simulink model "ModelOfTheRocket"  (R2020b)
settings: Solver=ode45  StartTime=0.0  StopTime=10  RelTol=1e-5
PostLoadFcn:
  | flightControlCallback('initializeParameters', bdroot, '3DOF', 0);
InitFcn:
  | flightControlCallback('runSim', bdroot);
libraries: aerolibasang x2, shared3dof x1, aerolibanim x1, simulink_extras x1
settings Model: Creator=yudan  LastModifiedBy=yudan
settings SolverCC: MinimalZcImpactIntegration=on
settings DataIOCC: ExternalInput=getinputstruct(op);  InitialState=getstatestruct(op);  SaveFormat=Array
settings OptimizationCC: EnhancedBackFolding=on  StrengthReduction=on  InitFltsAndDblsToZero=on  DifferentSizesBufferReuse=on
settings DebuggingCC: WriteAfterWriteMsg=DisableAll  AlgebraicLoopMsg=none  FcnCallInpInsideContextMsg=warning  UnconnectedInputMsg=none  UnconnectedOutputMsg=none  UnconnectedLineMsg=none  UniqueDataStoreMsg=error  StateNameClashWarn=warning  StrictBusMsg=ErrorOnBusTreatedAsVector  SFUnexpectedBacktrackingDiag=warning  SFNoUnconditionalDefaultTransitionDiag=warning  SFExecutionAtInitializationDiag=none  ArithmeticOperatorsInVariantConditions=warning
settings ModelReferenceCC: PropagateSignalLabelsOutOfModel=off
settings SFSimCC: SimUseLocalCustomCode=off
settings RTWCC: RTWUseLocalCustomCode=off
settings CodeAppCC: StateflowObjectComments=on

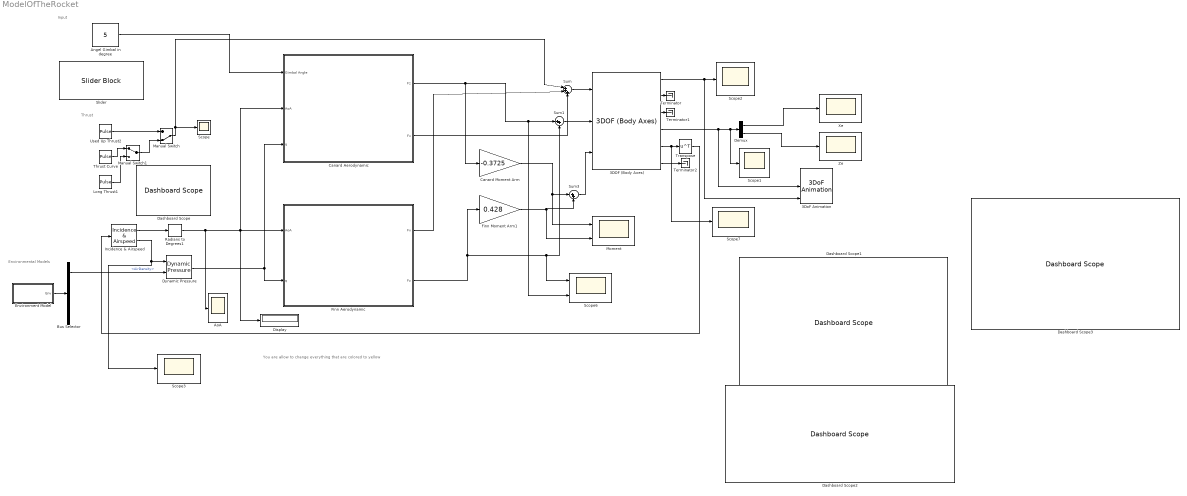
== system ModelOfTheRocket ==
  note: Input
  note: Thrust
  note: You are allow to change everything that are colored to yellow
  note: Environmental Models
  3DOF (Body Axes) : shared3dof/3DOF (Body Axes)  units=Metric (MKS)  mtype=Fixed  v_ini=100  theta_ini=0  alpha_ini=0  pos_ini=[0 0]  q_ini=0  mass=1.0  mass_e=0.5  mass_f=3.0  Iyy=1.0  Iyy_e=0.5  Iyy_f=3.0  g_in=Internal  g=9.81  vre_flag=on  abi_flag=off  aMode=0  vel_statename=''  theta_statename=''  pos_statename=''  q_statename=''  mass_statename=''
      settings: SourceProductBaseCode=AE,PW,MT,UV,VE,VP
  3DoF Animation : aerolibanim/3DoF Animation  u1=[-5000 5000 -2000 2000 -5000 5000]  u2=0.05  u3=2  u5=Fixed position  u6=[0 2000 0]  u7=10  u8=on
      settings: SourceProductBaseCode=AE
  Angel Gimbal in degree : Constant  Value=5
  AoA : Scope
  Bus Selector : BusSelector  OutputSignals=AirDensity,WindVelocity,g
  Canard Aerodynamic : Subsystem
  Canard Moment Arm : Gain  Description=Sign given by the normalized coordinate  Gain=-0.3725
  Dashboard Scope{,1..3} (4 alike) : DashboardScope
  Demux : Demux  Outputs=2
  Display : Display
  Dynamic Pressure : aerolibasang/Dynamic Pressure
  Environment Model : Subsystem  mask(Constant Environment Model){To=275.15, a=332.529, Po=79495.2, AirDensity=1.00649, ugvgwg=[-2 0 -1], pgqgrg=[0 0 0], g=[0 0 9.80665]}
      mask prompts: To "Constant Temperature (K):"; a "Constant Speed of Sound (m/s):"; Po "Constant Pressure (Pa):"; AirDensity "Constant Air Density (kg/m^3):"; ugvgwg "Constant Wind Velocity [ug vg wg] (m/s):"; pgqgrg "Constant Wind Angular Rates [pg qg rg] (rad/s):"; g "Constant Gravitational Acceleration (m/s^2):"
      mask Help: helpview(fullfile(docroot,'toolbox','aeroblks','aeroblks.map'), 'environment1');
      mask TypeOptions To: Constant Atmosphere/To
      mask TypeOptions a: Constant Atmosphere/a
      mask TypeOptions Po: Constant Atmosphere/Po
      mask TypeOptions AirDensity: Constant Atmosphere/AirDensity
      mask TypeOptions ugvgwg: Constant Wind/ugvgwg
      mask TypeOptions pgqgrg: Constant Wind/pgqgrg
      mask TypeOptions g: Constant Gravity/g
      mask DialogControl Container4 Prompt: Atmospheric Model
      mask DialogControl Container6 Prompt: Wind Model
      mask DialogControl Container8 Prompt: Gravity Model
      mask Display:
      | image('aeroenvironment.bmp','center')
      | port_label('output',1,'Env')
  Finn Aerodynamic : Subsystem
  Finn Moment Arm1 : Gain  Description=Sign given by the normalized coordinate  Gain=0.428
  Incidence & Airspeed : aerolibasang/Incidence  & Airspeed
      settings: SourceProductBaseCode=AE
  Long Thrust1 : DiscretePulseGenerator  PulseType=Time based  Amplitude=219  Period=1000  PulseWidth=99
  Manual Switch : ManualSwitch  CurrentSetting=0
  Manual Switch1 : ManualSwitch
  Moment : Scope  NumInputPorts=2
  Radians to Degrees1 : simulink_extras/Transformations/Radians to Degrees
  Scope{,1..3,7} (5 alike) : Scope
  Scope6 : Scope  NumInputPorts=2
  Slider : SliderBlock  ScaleMin=-5  ScaleMax=5
  Sum : Sum  Inputs=|+++
  Sum1 : Sum  Inputs=|++
  Sum3 : Sum  Inputs=|++
  Terminator : Terminator
  Terminator1 : Terminator
  Terminator2 : Terminator
  Thrust Curve : DiscretePulseGenerator  PulseType=Time based  Amplitude=219  Period=1000  PulseWidth=0.2
  Transpose : Math  Operator=transpose  SaturateOnIntegerOverflow=on
  Used Up Thrust2 : DiscretePulseGenerator  PulseType=Time based  Amplitude=0  Period=1000  PulseWidth=99
  Xe : Scope
  Ze : Scope
  wires:
  Sum/1 -> 3DOF (Body Axes)/1
  Sum1/1 -> 3DOF (Body Axes)/2
  Canard Moment Arm/1 -> Moment/1, Sum3/1
  Finn Moment Arm1/1 -> Moment/2, Sum3/2
  Dynamic Pressure/1 -> Canard Aerodynamic/3(q), Finn Aerodynamic/2(q)
  3DOF (Body Axes)/4 -> Scope1/1, Demux/1, 3DoF Animation/2
  3DOF (Body Axes)/1 -> 3DoF Animation/3, Scope2/1
  3DOF (Body Axes)/2 -> Terminator/1
  3DOF (Body Axes)/3 -> Terminator1/1
  3DOF (Body Axes)/6 -> Terminator2/1
  Incidence & Airspeed/2 -> Scope3/1, Dynamic Pressure/1
  3DOF (Body Axes)/5 -> Scope7/1, Transpose/1
  Transpose/1 -> Incidence & Airspeed/1
  Demux/1 -> Xe/1
  Demux/2 -> Ze/1
  Manual Switch/1 -> Sum/1, Scope/1
  Used Up Thrust2/1 -> Manual Switch/1
  Canard Aerodynamic/1(Fz) -> Canard Moment Arm/1, Scope6/2, Sum1/1
  Canard Aerodynamic/2(Fx) -> Sum/3
  Finn Aerodynamic/2(Fz) -> Finn Moment Arm1/1, Scope6/1, Sum1/2
  Finn Aerodynamic/1(Fx) -> Sum/2
  Angel Gimbal in degree/1 -> Canard Aerodynamic/1(Gimbal Angle)
  Incidence & Airspeed/1 -> Radians to Degrees1/1
  Sum3/1 -> 3DOF (Body Axes)/3
  Radians to Degrees1/1 -> Finn Aerodynamic/1(AoA), Canard Aerodynamic/2(AoA), Display/1, AoA/1
  Manual Switch1/1 -> Manual Switch/2
  Thrust Curve/1 -> Manual Switch1/1
  Long Thrust1/1 -> Manual Switch1/2
  Environment Model/1(Env) -> Bus Selector/1
  Bus Selector/1 -> Dynamic Pressure/2  "<AirDensity>"

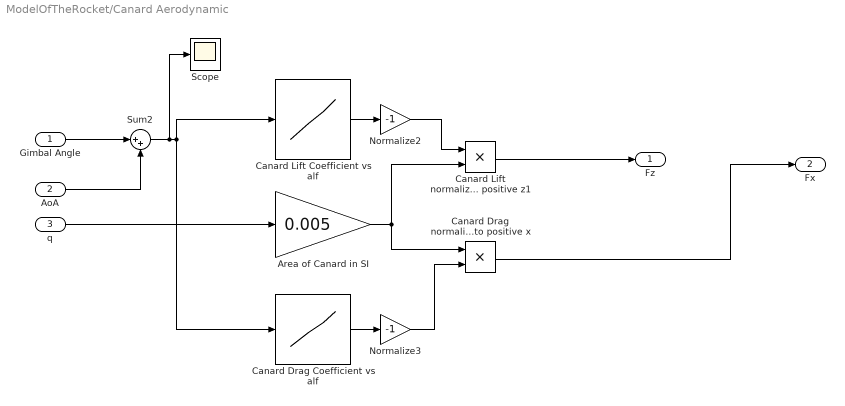
== system ModelOfTheRocket/Canard Aerodynamic ==
  Gimbal Angle : Inport
  AoA : Inport  Port=2
  q : Inport  Port=3
  Area of Canard in SI : Gain  Gain=0.005
  Canard Drag Coefficient vs alf : Lookup_n-D  NumberOfTableDimensions=1  BreakpointsForDimension1=|  Table=|  InternalRulePriority=Speed  RndMeth=Simplest  InputSameDT=on
      BreakpointsForDimension1=|
      | [-6
      | -5.9
      | -5.8
      | -5.7
      | -5.6
      | -5.5
      | -5.4
      | -5.3
      | -5.2
      | -5.1
      | -5
      | -4.9
      | -4.8
      | -4.7
      | -4.6
      | -4.5
      | -4.4
      | -4.3
      | -4.2
      | -4.1
      | -4
      | -3.9
      | -3.8
      | -3.7
      | -3.6
      | -3.5
      | -3.4
      | -3.3
      | -3.2
      | -3.1
      | -3
      | -2.9
      | -2.8
      | -2.7
      | -2.6
      | -2.4
      | -2.3
      | -2.2
      | -2.1
      | -2
      | -1.9
      | -1.8
      | -1.7
      | -1.6
      | -1.5
      | -1.4
      | -1.3
      | -1.2
      | -1.1
      | -1
      | -0.9
      | -0.8
      | -0.7
      | -0.6
      | -0.5
      | -0.4
      | -0.3
      | -0.2
      | -0.1
      | 0
      | 0.1
      | 0.2
      | 0.3
      | 0.4
      | 0.5
      | 0.6
      | 0.7
      | 0.8
      | 0.9
      | 1
      | 1.1
      | 1.2
      | 1.3
      | 1.4
      | 1.5
      | 1.6
      | 1.7
      | 1.8
      | 1.9
      | 2
      | 2.1
      | 2.2
      | 2.3
      | 2.4
      | 2.5
      | 2.6
      | 2.7
      | 2.8
      | 2.9
      | 3
      | 3.1
      | 3.2
      | 3.3
      | 3.4
      | 3.5
      | 3.6
      | 3.7
      | 3.8
      | 3.9
      | 4
      | 4.1
      | 4.2
      | 4.3
      | 4.4
      | 4.5
      | 4.6
      | 4.7
      | 4.8
      | 4.9
      | 5
      | 5.1
      | 5.2
      | 5.3
      | 5.4
      | 5.5
      | 5.6
      | 5.7
      | 5.8
      | 5.9
      | 6]
      Table=|
      | [0.04364
      | 0.04148
      | 0.03935
      | 0.03724
      | 0.03517
      | 0.03314
      | 0.03118
      | 0.02935
      | 0.02764
      | 0.02597
      | 0.02431
      | 0.02272
      | 0.02125
      | 0.01988
      | 0.01863
      | 0.01752
      | 0.01655
      | 0.01573
      | 0.01489
      | 0.01373
      | 0.01297
      | 0.01255
      | 0.01218
      | 0.01173
      | 0.0113
      | 0.01092
      | 0.01063
      | 0.01009
      | 0.0098
      | 0.0096
      | 0.00942
      | 0.00909
      | 0.00891
      | 0.00868
      | 0.00844
      | 0.00786
      | 0.00753
      | 0.00719
      | 0.00689
      | 0.00663
      | 0.00637
      | 0.00613
      | 0.00593
      | 0.00573
      | 0.00555
      | 0.00538
      | 0.00522
      | 0.00508
      | 0.00495
      | 0.00484
      | 0.00475
      | 0.00469
      | 0.00465
      | 0.00462
      | 0.00462
      | 0.00463
      | 0.00464
      | 0.00465
      | 0.00465
      | 0.00465
      | 0.00465
      | 0.00465
      | 0.00464
      | 0.00463
      | 0.00462
      | 0.00462
      | 0.00465
      | 0.00469
      | 0.00475
      | 0.00484
      | 0.00495
      | 0.00508
      | 0.00522
      | 0.00538
      | 0.00555
      | 0.00573
      | 0.00593
      | 0.00613
      | 0.00637
      | 0.00663
      | 0.00689
      | 0.00719
      | 0.00752
      | 0.00786
      | 0.00817
      | 0.00844
      | 0.00868
      | 0.00891
      | 0.00908
      | 0.00942
      | 0.00961
      | 0.0098
      | 0.01008
      | 0.01063
      | 0.01092
      | 0.0113
      | 0.01173
      | 0.01217
      | 0.01254
      | 0.01297
      | 0.01373
      | 0.0149
      | 0.01572
      | 0.01655
      | 0.01752
      | 0.01863
      | 0.01988
      | 0.02125
      | 0.02273
      | 0.02432
      | 0.02598
      | 0.02764
      | 0.02935
      | 0.03119
      | 0.03316
      | 0.03518
      | 0.03725
      | 0.03936
      | 0.0415
      | 0.04366
      | ]
  Canard Drag normalized to positive x : Product
  Canard Lift Coefficient vs alf : Lookup_n-D  NumberOfTableDimensions=1  BreakpointsForDimension1=|  Table=|  InternalRulePriority=Speed  RndMeth=Simplest  InputSameDT=on
      BreakpointsForDimension1=|
      | [-6
      | -5.9
      | -5.8
      | -5.7
      | -5.6
      | -5.5
      | -5.4
      | -5.3
      | -5.2
      | -5.1
      | -5
      | -4.9
      | -4.8
      | -4.7
      | -4.6
      | -4.5
      | -4.4
      | -4.3
      | -4.2
      | -4.1
      | -4
      | -3.9
      | -3.8
      | -3.7
      | -3.6
      | -3.5
      | -3.4
      | -3.3
      | -3.2
      | -3.1
      | -3
      | -2.9
      | -2.8
      | -2.7
      | -2.6
      | -2.4
      | -2.3
      | -2.2
      | -2.1
      | -2
      | -1.9
      | -1.8
      | -1.7
      | -1.6
      | -1.5
      | -1.4
      | -1.3
      | -1.2
      | -1.1
      | -1
      | -0.9
      | -0.8
      | -0.7
      | -0.6
      | -0.5
      | -0.4
      | -0.3
      | -0.2
      | -0.1
      | 0
      | 0.1
      | 0.2
      | 0.3
      | 0.4
      | 0.5
      | 0.6
      | 0.7
      | 0.8
      | 0.9
      | 1
      | 1.1
      | 1.2
      | 1.3
      | 1.4
      | 1.5
      | 1.6
      | 1.7
      | 1.8
      | 1.9
      | 2
      | 2.1
      | 2.2
      | 2.3
      | 2.4
      | 2.5
      | 2.6
      | 2.7
      | 2.8
      | 2.9
      | 3
      | 3.1
      | 3.2
      | 3.3
      | 3.4
      | 3.5
      | 3.6
      | 3.7
      | 3.8
      | 3.9
      | 4
      | 4.1
      | 4.2
      | 4.3
      | 4.4
      | 4.5
      | 4.6
      | 4.7
      | 4.8
      | 4.9
      | 5
      | 5.1
      | 5.2
      | 5.3
      | 5.4
      | 5.5
      | 5.6
      | 5.7
      | 5.8
      | 5.9
      | 6]
      Table=|
      | [-0.6705
      | -0.6674
      | -0.6637
      | -0.6595
      | -0.6547
      | -0.6492
      | -0.6428
      | -0.6357
      | -0.628
      | -0.6204
      | -0.6127
      | -0.6045
      | -0.5957
      | -0.5863
      | -0.5762
      | -0.5657
      | -0.5547
      | -0.5432
      | -0.5319
      | -0.5218
      | -0.5109
      | -0.4992
      | -0.4873
      | -0.4757
      | -0.4642
      | -0.4525
      | -0.4407
      | -0.43
      | -0.4184
      | -0.4064
      | -0.3945
      | -0.383
      | -0.3711
      | -0.3595
      | -0.3479
      | -0.3254
      | -0.3144
      | -0.3035
      | -0.2924
      | -0.2812
      | -0.27
      | -0.2588
      | -0.2475
      | -0.2363
      | -0.2251
      | -0.2139
      | -0.2027
      | -0.1916
      | -0.1806
      | -0.1698
      | -0.1592
      | -0.1488
      | -0.1369
      | -0.1201
      | -0.1027
      | -0.0839
      | -0.0632
      | -0.0417
      | -0.0212
      | 0
      | 0.0212
      | 0.0417
      | 0.0633
      | 0.0839
      | 0.1027
      | 0.1202
      | 0.137
      | 0.1487
      | 0.1591
      | 0.1698
      | 0.1806
      | 0.1916
      | 0.2026
      | 0.2138
      | 0.225
      | 0.2362
      | 0.2475
      | 0.2588
      | 0.27
      | 0.2811
      | 0.2923
      | 0.3034
      | 0.3144
      | 0.3253
      | 0.3365
      | 0.3479
      | 0.3594
      | 0.3711
      | 0.383
      | 0.3944
      | 0.4064
      | 0.4183
      | 0.4299
      | 0.4406
      | 0.4525
      | 0.4641
      | 0.4756
      | 0.4873
      | 0.4992
      | 0.5109
      | 0.5218
      | 0.5319
      | 0.5433
      | 0.5547
      | 0.5657
      | 0.5763
      | 0.5863
      | 0.5958
      | 0.6046
      | 0.6128
      | 0.6204
      | 0.6281
      | 0.6358
      | 0.643
      | 0.6493
      | 0.6548
      | 0.6596
      | 0.6638
      | 0.6675
      | 0.6706]
  Canard Lift normalized to positive z1 : Product
  Normalize2 : Gain  Gain=-1
  Normalize3 : Gain  Gain=-1
  Scope : Scope
  Sum2 : Sum  Inputs=|++
  Fz : Outport
  Fx : Outport  Port=2
  wires:
  Area of Canard in SI/1 -> Canard Drag normalized to positive x/1, Canard Lift normalized to positive z1/2
  Canard Drag Coefficient vs alf/1 -> Normalize3/1
  Canard Drag normalized to positive x/1 -> Fx/1
  Normalize2/1 -> Canard Lift normalized to positive z1/1
  Sum2/1 -> Scope/1, Canard Drag Coefficient vs alf/1, Canard Lift Coefficient vs alf/1
  Normalize3/1 -> Canard Drag normalized to positive x/2
  Canard Lift Coefficient vs alf/1 -> Normalize2/1
  Canard Lift normalized to positive z1/1 -> Fz/1
  Gimbal Angle/1 -> Sum2/1
  q/1 -> Area of Canard in SI/1
  AoA/1 -> Sum2/2

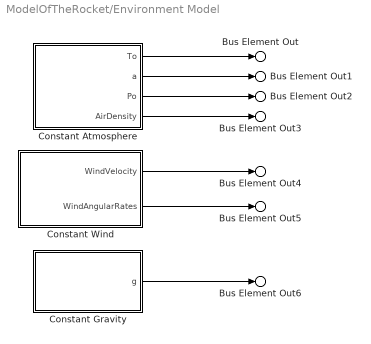
== system ModelOfTheRocket/Environment Model ==
  Constant Atmosphere : Subsystem  VariantControl=atmosCONST  mask(Standard Atmospheric Constants){To=To, a=a, Po=Po, AirDensity=AirDensity}
      mask prompts: To "Constant Temperature (K):"; a "Constant Speed of Sound (m/s):"; Po "Constant Pressure (Pa):"; AirDensity "Constant Air Density (kg/m^3):"
  Constant Gravity : Subsystem  VariantControl=gravCONST  mask(Constant Gravitational Acceleration){g=g}
      mask prompts: g "Constant Gravitational Acceleration (m/s^2):"
  Constant Wind : Subsystem  VariantControl=windCONST  mask(Constant Wind Values){ugvgwg=ugvgwg, pgqgrg=pgqgrg}
      mask prompts: ugvgwg "Constant Wind Velocity (m/s):"; pgqgrg "Constant Wind Angular Rates (rad/s):"
  Bus Element Out : Outport  VectorParamsAs1DForOutWhenUnconnected=off  PortName=Env  Element=To
  Bus Element Out1 : Outport  VectorParamsAs1DForOutWhenUnconnected=off  PortName=Env  Element=a
  Bus Element Out2 : Outport  VectorParamsAs1DForOutWhenUnconnected=off  PortName=Env  Element=Po
  Bus Element Out3 : Outport  VectorParamsAs1DForOutWhenUnconnected=off  PortName=Env  Element=AirDensity
  Bus Element Out4 : Outport  VectorParamsAs1DForOutWhenUnconnected=off  PortName=Env  Element=WindVelocity
  Bus Element Out5 : Outport  VectorParamsAs1DForOutWhenUnconnected=off  PortName=Env  Element=WindAngularRates
  Bus Element Out6 : Outport  VectorParamsAs1DForOutWhenUnconnected=off  PortName=Env  Element=g
  wires:
  Constant Gravity/1(g) -> Bus Element Out6/1
  Constant Atmosphere/2(a) -> Bus Element Out1/1
  Constant Wind/1(WindVelocity) -> Bus Element Out4/1
  Constant Atmosphere/1(To) -> Bus Element Out/1
  Constant Atmosphere/4(AirDensity) -> Bus Element Out3/1
  Constant Atmosphere/3(Po) -> Bus Element Out2/1
  Constant Wind/2(WindAngularRates) -> Bus Element Out5/1

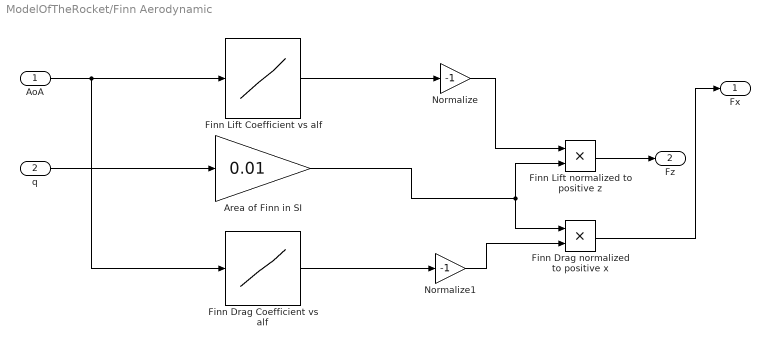
== system ModelOfTheRocket/Finn Aerodynamic ==
  AoA : Inport
  q : Inport  Port=2
  Area of Finn in SI : Gain  Gain=0.01
  Finn Drag Coefficient vs alf : Lookup_n-D  NumberOfTableDimensions=1  BreakpointsForDimension1=|  Table=|  InternalRulePriority=Speed  RndMeth=Simplest  InputSameDT=on
      BreakpointsForDimension1=|
      | [-6.8
      | -6.7
      | -6.6
      | -6.5
      | -6.4
      | -6.3
      | -6.2
      | -6.1
      | -6
      | -5.9
      | -5.8
      | -5.7
      | -5.6
      | -5.5
      | -5.4
      | -5.3
      | -5.2
      | -5.1
      | -5
      | -4.9
      | -4.8
      | -4.7
      | -4.6
      | -4.5
      | -4.4
      | -4.3
      | -4.2
      | -4.1
      | -4
      | -3.9
      | -3.8
      | -3.7
      | -3.6
      | -3.5
      | -3.4
      | -3.3
      | -3.2
      | -3.1
      | -3
      | -2.9
      | -2.8
      | -2.7
      | -2.6
      | -2.5
      | -2.4
      | -2.3
      | -2.2
      | -2.1
      | -2
      | -1.9
      | -1.8
      | -1.7
      | -1.6
      | -1.5
      | -1.4
      | -1.3
      | -1.2
      | -1.1
      | -1
      | -0.9
      | -0.8
      | -0.7
      | -0.6
      | -0.3
      | -0.2
      | -0.1
      | 0
      | 0.1
      | 0.2
      | 0.3
      | 0.4
      | 0.5
      | 0.6
      | 0.7
      | 0.8
      | 0.9
      | 1
      | 1.1
      | 1.2
      | 1.3
      | 1.4
      | 1.5
      | 1.6
      | 1.7
      | 1.8
      | 1.9
      | 2
      | 2.1
      | 2.2
      | 2.3
      | 2.4
      | 2.5
      | 2.6
      | 2.7
      | 2.8
      | 2.9
      | 3
      | 3.1
      | 3.2
      | 3.3
      | 3.4
      | 3.5
      | 3.6
      | 3.7
      | 3.8
      | 3.9
      | 4
      | 4.1
      | 4.2
      | 4.3
      | 4.4
      | 4.5
      | 4.6
      | 4.7
      | 4.8
      | 4.9
      | 5
      | 5.1
      | 5.2
      | 5.3
      | 5.4
      | 5.5
      | 5.6
      | 5.7
      | 5.8
      | 5.9
      | 6
      | 6.1
      | 6.2
      | 6.3
      | 6.4
      | 6.5
      | 6.6
      | 6.7
      | 6.8
      | 6.9
      | 7
      | ]
      Table=|
      | [ 0.06066
      | 0.05792
      | 0.05522
      | 0.05254
      | 0.04988
      | 0.04725
      | 0.04464
      | 0.0421
      | 0.03963
      | 0.03724
      | 0.03493
      | 0.03273
      | 0.03061
      | 0.02859
      | 0.02663
      | 0.02474
      | 0.02296
      | 0.02123
      | 0.0196
      | 0.01808
      | 0.01669
      | 0.01561
      | 0.0146
      | 0.01369
      | 0.01283
      | 0.01212
      | 0.01154
      | 0.01107
      | 0.01018
      | 0.00972
      | 0.0094
      | 0.00913
      | 0.00889
      | 0.0087
      | 0.00854
      | 0.00827
      | 0.00799
      | 0.00784
      | 0.00771
      | 0.00761
      | 0.00741
      | 0.00731
      | 0.00716
      | 0.00703
      | 0.00689
      | 0.00671
      | 0.00652
      | 0.00632
      | 0.00611
      | 0.00585
      | 0.00561
      | 0.0054
      | 0.00518
      | 0.00499
      | 0.00482
      | 0.00464
      | 0.00448
      | 0.00433
      | 0.00419
      | 0.00406
      | 0.00394
      | 0.00383
      | 0.00373
      | 0.00352
      | 0.00348
      | 0.00346
      | 0.00345
      | 0.00346
      | 0.00348
      | 0.00352
      | 0.00357
      | 0.00365
      | 0.00373
      | 0.00383
      | 0.00394
      | 0.00406
      | 0.00419
      | 0.00433
      | 0.00448
      | 0.00464
      | 0.00482
      | 0.00499
      | 0.00519
      | 0.0054
      | 0.00561
      | 0.00585
      | 0.00611
      | 0.00632
      | 0.00652
      | 0.00671
      | 0.00689
      | 0.00703
      | 0.00716
      | 0.00731
      | 0.00741
      | 0.00761
      | 0.0077
      | 0.00784
      | 0.00799
      | 0.00827
      | 0.00854
      | 0.0087
      | 0.00889
      | 0.00913
      | 0.0094
      | 0.00971
      | 0.01018
      | 0.01107
      | 0.01154
      | 0.01211
      | 0.01283
      | 0.01369
      | 0.01461
      | 0.01559
      | 0.01671
      | 0.01808
      | 0.01961
      | 0.02124
      | 0.02295
      | 0.02475
      | 0.02662
      | 0.02858
      | 0.03062
      | 0.03274
      | 0.03494
      | 0.03724
      | 0.03964
      | 0.04212
      | 0.04465
      | 0.04727
      | 0.0499
      | 0.05256
      | 0.05525
      | 0.05796
      | 0.06068
      | 0.06346
      | 0.06618
      | 
      | ]
  Finn Drag normalized to positive x : Product
  Finn Lift Coefficient vs alf : Lookup_n-D  NumberOfTableDimensions=1  BreakpointsForDimension1=|  Table=|  InternalRulePriority=Speed  RndMeth=Simplest  InputSameDT=on
      BreakpointsForDimension1=|
      | [-6.8
      | -6.7
      | -6.6
      | -6.5
      | -6.4
      | -6.3
      | -6.2
      | -6.1
      | -6
      | -5.9
      | -5.8
      | -5.7
      | -5.6
      | -5.5
      | -5.4
      | -5.3
      | -5.2
      | -5.1
      | -5
      | -4.9
      | -4.8
      | -4.7
      | -4.6
      | -4.5
      | -4.4
      | -4.3
      | -4.2
      | -4.1
      | -4
      | -3.9
      | -3.8
      | -3.7
      | -3.6
      | -3.5
      | -3.4
      | -3.3
      | -3.2
      | -3.1
      | -3
      | -2.9
      | -2.8
      | -2.7
      | -2.6
      | -2.5
      | -2.4
      | -2.3
      | -2.2
      | -2.1
      | -2
      | -1.9
      | -1.8
      | -1.7
      | -1.6
      | -1.5
      | -1.4
      | -1.3
      | -1.2
      | -1.1
      | -1
      | -0.9
      | -0.8
      | -0.7
      | -0.6
      | -0.3
      | -0.2
      | -0.1
      | 0
      | 0.1
      | 0.2
      | 0.3
      | 0.4
      | 0.5
      | 0.6
      | 0.7
      | 0.8
      | 0.9
      | 1
      | 1.1
      | 1.2
      | 1.3
      | 1.4
      | 1.5
      | 1.6
      | 1.7
      | 1.8
      | 1.9
      | 2
      | 2.1
      | 2.2
      | 2.3
      | 2.4
      | 2.5
      | 2.6
      | 2.7
      | 2.8
      | 2.9
      | 3
      | 3.1
      | 3.2
      | 3.3
      | 3.4
      | 3.5
      | 3.6
      | 3.7
      | 3.8
      | 3.9
      | 4
      | 4.1
      | 4.2
      | 4.3
      | 4.4
      | 4.5
      | 4.6
      | 4.7
      | 4.8
      | 4.9
      | 5
      | 5.1
      | 5.2
      | 5.3
      | 5.4
      | 5.5
      | 5.6
      | 5.7
      | 5.8
      | 5.9
      | 6
      | 6.1
      | 6.2
      | 6.3
      | 6.4
      | 6.5
      | 6.6
      | 6.7
      | 6.8
      | 6.9
      | 7
      | ]
      Table=|
      | [-0.6956
      | -0.6951
      | -0.6945
      | -0.6938
      | -0.6927
      | -0.6914
      | -0.6896
      | -0.6873
      | -0.6845
      | -0.681
      | -0.6769
      | -0.6723
      | -0.667
      | -0.6611
      | -0.6548
      | -0.6479
      | -0.6405
      | -0.6326
      | -0.6241
      | -0.6152
      | -0.6057
      | -0.5952
      | -0.5844
      | -0.5734
      | -0.5622
      | -0.5509
      | -0.5393
      | -0.5275
      | -0.5175
      | -0.5062
      | -0.4944
      | -0.4824
      | -0.4705
      | -0.4584
      | -0.4463
      | -0.4346
      | -0.4229
      | -0.4109
      | -0.3988
      | -0.3867
      | -0.3749
      | -0.3629
      | -0.3511
      | -0.3393
      | -0.3276
      | -0.316
      | -0.3045
      | -0.293
      | -0.2799
      | -0.2637
      | -0.2475
      | -0.231
      | -0.2152
      | -0.1994
      | -0.1831
      | -0.1667
      | -0.1505
      | -0.1362
      | -0.1208
      | -0.1061
      | -0.092
      | -0.0785
      | -0.0655
      | -0.0315
      | -0.0209
      | -0.0104
      | 0
      | 0.0104
      | 0.0209
      | 0.0315
      | 0.0424
      | 0.0536
      | 0.0655
      | 0.0785
      | 0.092
      | 0.1062
      | 0.1208
      | 0.1362
      | 0.1505
      | 0.1667
      | 0.1831
      | 0.1994
      | 0.2152
      | 0.231
      | 0.2476
      | 0.2638
      | 0.2799
      | 0.2929
      | 0.3045
      | 0.316
      | 0.3275
      | 0.3392
      | 0.351
      | 0.3628
      | 0.3748
      | 0.3866
      | 0.3987
      | 0.4108
      | 0.4228
      | 0.4345
      | 0.4462
      | 0.4583
      | 0.4704
      | 0.4824
      | 0.4943
      | 0.5062
      | 0.5175
      | 0.5275
      | 0.5393
      | 0.5509
      | 0.5622
      | 0.5734
      | 0.5844
      | 0.5952
      | 0.6056
      | 0.6152
      | 0.6242
      | 0.6326
      | 0.6405
      | 0.6479
      | 0.6549
      | 0.6612
      | 0.6671
      | 0.6724
      | 0.6771
      | 0.6811
      | 0.6846
      | 0.6874
      | 0.6898
      | 0.6915
      | 0.6929
      | 0.6939
      | 0.6947
      | 0.6953
      | 0.6958
      | 0.6963
      | 0.6957
      | ]
  Finn Lift normalized to positive z : Product
  Normalize : Gain  Gain=-1
  Normalize1 : Gain  Gain=-1
  Fx : Outport
  Fz : Outport  Port=2
  wires:
  Finn Lift normalized to positive z/1 -> Fz/1
  Finn Drag normalized to positive x/1 -> Fx/1
  Normalize1/1 -> Finn Drag normalized to positive x/2
  Finn Lift Coefficient vs alf/1 -> Normalize/1
  Normalize/1 -> Finn Lift normalized to positive z/1
  Area of Finn in SI/1 -> Finn Drag normalized to positive x/1, Finn Lift normalized to positive z/2
  Finn Drag Coefficient vs alf/1 -> Normalize1/1
  q/1 -> Area of Finn in SI/1
  AoA/1 -> Finn Drag Coefficient vs alf/1, Finn Lift Coefficient vs alf/1

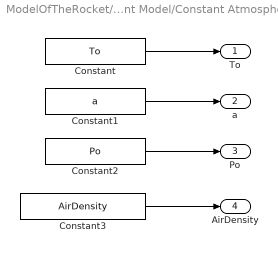
== system ModelOfTheRocket/Environment Model/Constant Atmosphere ==
  Constant : Constant  Value=To
  Constant1 : Constant  Value=a
  Constant2 : Constant  Value=Po
  Constant3 : Constant  Value=AirDensity
  To : Outport  VectorParamsAs1DForOutWhenUnconnected=off
  a : Outport  Port=2  VectorParamsAs1DForOutWhenUnconnected=off
  Po : Outport  Port=3  VectorParamsAs1DForOutWhenUnconnected=off
  AirDensity : Outport  Port=4  VectorParamsAs1DForOutWhenUnconnected=off
  wires:
  Constant3/1 -> AirDensity/1
  Constant2/1 -> Po/1
  Constant/1 -> To/1
  Constant1/1 -> a/1

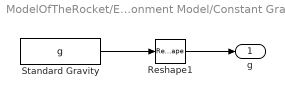
== system ModelOfTheRocket/Environment Model/Constant Gravity ==
  Reshape1 : Reshape  OutputDimensionality=Column vector (2-D)
  Standard Gravity : Constant  Value=g
  g : Outport  VectorParamsAs1DForOutWhenUnconnected=off
  wires:
  Standard Gravity/1 -> Reshape1/1
  Reshape1/1 -> g/1

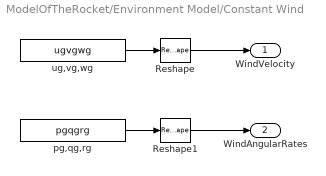
== system ModelOfTheRocket/Environment Model/Constant Wind ==
  Reshape : Reshape  OutputDimensionality=Column vector (2-D)
  Reshape1 : Reshape  OutputDimensionality=Column vector (2-D)
  pg,qg,rg : Constant  Value=pgqgrg
  ug,vg,wg : Constant  Value=ugvgwg
  WindVelocity : Outport  VectorParamsAs1DForOutWhenUnconnected=off
  WindAngularRates : Outport  Port=2  VectorParamsAs1DForOutWhenUnconnected=off
  wires:
  Reshape1/1 -> WindAngularRates/1
  Reshape/1 -> WindVelocity/1
  ug,vg,wg/1 -> Reshape/1
  pg,qg,rg/1 -> Reshape1/1
